simulink model "Build"  (R2016b)
settings: Solver=FixedStepDiscrete  StartTime=0.0  StopTime=10.0  RelTol=1e-3
settings Model: Creator=3essawy  LastModifiedBy=3essawy
settings OptimizationCC: DefaultParameterBehavior=Inlined
settings DebuggingCC: ParameterTunabilityLossMsg=error
settings SFSimCC: SimCustomSourceCode=|
  | led.c
  | Switch.c
settings SFSimCC: SimCustomHeaderCode=|
  | #include"led.h"
  | #include"Switch.h"
settings SFSimCC: SimUserSources=|
  | led.c
  | Switch.c
settings RTWCC: SystemTargetFile=ert.tlc  GenCodeOnly=on  TemplateMakefile=ert_default_tmf  Description=Embedded Coder  GenerateReport=on  RTWUseSimCustomCode=on  IncludeHyperlinkInReport=on  LaunchReport=on  GenerateTraceInfo=on  GenerateTraceReport=on  GenerateTraceReportSl=on  GenerateTraceReportSf=on  GenerateTraceReportEml=on
settings RTWCC: CustomSourceCode=|
  | led.c
  | Switch.c
settings RTWCC: CustomHeaderCode=|
  | #include"led.h"
  | #include"Switch.h"
settings RTWCC: CustomSource=|
  | led.c
  | Switch.c
settings CodeAppCC: ForceParamTrailComments=on  IgnoreCustomStorageClasses=off  OperatorAnnotations=on  SimulinkDataObjDesc=on  SFDataObjDesc=on  MATLABFcnDesc=on  InsertBlockDesc=on  MATLABSourceComments=on
settings ERTTargetCC: TargetLangStandard=C99 (ISO)  GenerateSampleERTMain=on  InlinedParameterPlacement=NonHierarchical  ERTCustomFileTemplate=example_file_process.tlc  EnableUserReplacementTypes=on

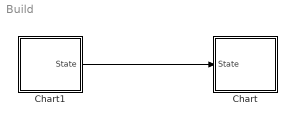
== system Build ==
  Chart : Stateflow chart  TreatAsAtomicUnit=on
  Chart1 : Stateflow chart  TreatAsAtomicUnit=on
  wires:
  Chart1/1(State) -> Chart/1(State)

== stateflow chart Build/Chart1 ==
  (default) -> (junction 7) : {Res=ChechState();}
  (junction 7) -> (junction 8) [order 1] : [Res==1]
  (junction 7) -> (junction 9) [order 2] : {State=0;}
  (junction 8) -> (junction 10) : {State=1;}
  (junction 10) -> (junction 9)
  (junction 9) -> (junction 11)
  data: State output uint32; Res local double

== stateflow chart Build/Chart ==
  (default) -> (junction 11)
  (junction 11) -> (junction 12) [order 1] : [State==1]
  (junction 11) -> (junction 13) [order 2] : {led_off(led_id0);}
  (junction 12) -> (junction 14) : {led_on(led_id0);}
  (junction 14) -> (junction 13)
  (junction 13) -> (junction 15)
  data: State input uint32
